simulink model "Observador_de_Estados_Simulink2016b"  (R2016b)
settings: Solver=VariableStepAuto  StartTime=0.0  StopTime=10.0  RelTol=1e-3
values from neighbouring files (symbols this model uses):
  A = [0 1;      1000 0]    [LIST3_Q5_a.m]    (also in LIST3_Q5_b.m)
  B = [0;      20]    [LIST3_Q5_a.m]    (also in LIST3_Q5_b.m)
  C = [1 3]    [LIST3_Q2.m]    (also in LIST3_Q5_a.m = SS2_z.C; LIST3_Q5_b.m = SS2_z.C; LIST3_Q6_a.m = [1 0]; LIST3_Q6_b.m = [1 0])
  L = [L1; L2]    [LIST3_Q4.m]    (also in LIST3_Q6_c.m = Lt')
undefined symbols (not defined in the file or in its folder): T, xo_1
settings Model: Creator=ribei  LastModifiedBy=ribei
settings DataIOCC: ReturnWorkspaceOutputs=on
settings DebuggingCC: UnconnectedInputMsg=none  UnconnectedOutputMsg=none  UnconnectedLineMsg=none
settings ModelReferenceCC: EnableRefExpFcnMdlSchedulingChecks=off
settings SFSimCC: SimUseLocalCustomCode=on
settings RTWCC: RTWUseLocalCustomCode=on

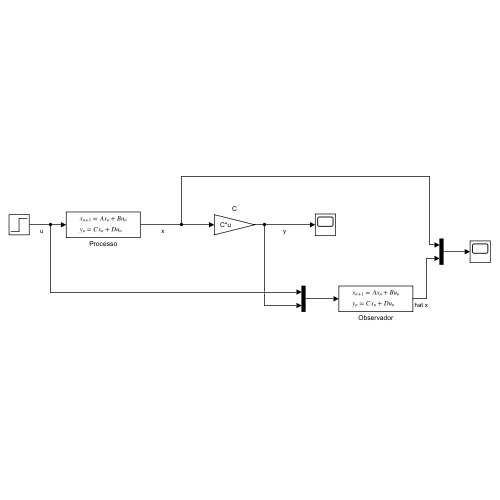
[thumbnail: Simulink's stored preview of the top-level diagram]
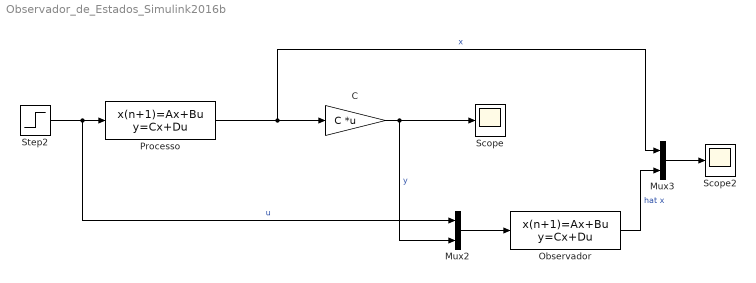
== system Observador_de_Estados_Simulink2016b ==
  C : Gain  Gain=C  Multiplication=Matrix(K*u)
  Mux2 : Mux  Inputs=2
  Mux3 : Mux  Inputs=2
  Observador : DiscreteStateSpace  A=(A-L*C)  B=[B L]  C=eye(2)  D=zeros(2,2)  X0=[0;0]  SampleTime=T
  Processo : DiscreteStateSpace  A=A  B=B  C=eye(2)  D=zeros(2,1)  X0=xo_1  SampleTime=T
  Scope : Scope
  Scope2 : Scope
  Step2 : Step  SampleTime=0
  wires:
  Processo/1 -> Mux3/1, C/1  "x"
  C/1 -> Mux2/2, Scope/1  "y"
  Step2/1 -> Mux2/1, Processo/1  "u"
  Mux2/1 -> Observador/1
  Observador/1 -> Mux3/2  "hat x"
  Mux3/1 -> Scope2/1
